simulink library "x2qqp"  (R2023a)
settings: Solver=VariableStepAuto  StartTime=0.0  StopTime=10.0  RelTol=1e-3
settings Model: Creator=pinki  LastModifiedBy=pinki

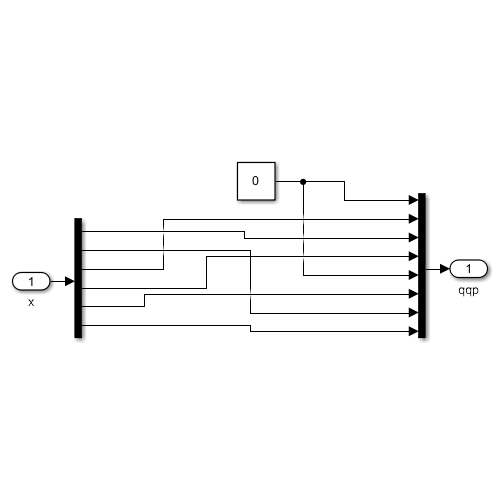
[thumbnail: Simulink's stored preview of the top-level diagram]
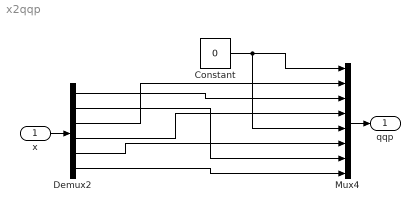
== system x2qqp ==
  x : Inport
  Constant : Constant  Value=0
  Demux2 : Demux  Outputs=6
  Mux4 : Mux  Inputs=8
  qqp : Outport
  wires:
  Demux2/6 -> Mux4/8
  Mux4/1 -> qqp/1
  x/1 -> Demux2/1
  Demux2/3 -> Mux4/2
  Demux2/1 -> Mux4/3
  Demux2/5 -> Mux4/6
  Demux2/4 -> Mux4/4
  Constant/1 -> Mux4/1, Mux4/5
  Demux2/2 -> Mux4/7
